simulink model "modelo_SIS"  (R2019b)
settings: Solver=VariableStepAuto  StartTime=0.0  StopTime=500  RelTol=1e-3
settings Model: Creator=lucia  LastModifiedBy=lucia

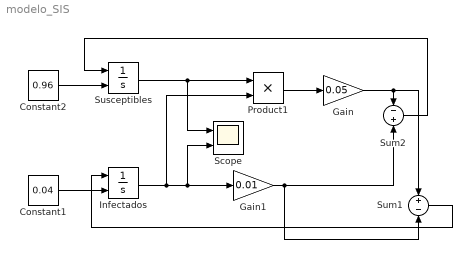
== system modelo_SIS ==
  Constant1 : Constant  Value=0.04
  Constant2 : Constant  Value=0.96
  Gain : Gain  Gain=0.05
  Gain1 : Gain  Gain=0.01
  Infectados : Integrator  InitialConditionSource=external
  Product1 : Product
  Scope : Scope  NumInputPorts=2
  Sum1 : Sum  Inputs=+-
  Sum2 : Sum  Inputs=-+
  Susceptibles : Integrator  InitialConditionSource=external
  wires:
  Constant2/1 -> Susceptibles/2
  Constant1/1 -> Infectados/2
  Susceptibles/1 -> Scope/1, Product1/1
  Infectados/1 -> Product1/2, Scope/2, Gain1/1
  Product1/1 -> Gain/1
  Gain/1 -> Sum1/1, Sum2/1
  Gain1/1 -> Sum1/2, Sum2/2
  Sum2/1 -> Susceptibles/1
  Sum1/1 -> Infectados/1
